simulink model "gm_mandelbrot_fpga"  (R2019b)
settings: Solver=FixedStepDiscrete  StartTime=0.0  StopTime=33.5e-3  FixedStep=0.5*Ts  RelTol=1e-3  EnableMultiTasking=on
undefined symbols (not defined in the file or in its folder): BUTTON_CLOCK_DIV, BUTTON_DEBOUNCE, BUTTON_POLLING, LUT_BLUE, LUT_GREEN, LUT_RED, MAX_ITERATIONS, PIXEL_TIME, TRASLATION_FACTOR, Ts, VGA_HORIZONTAL_BACK_PORCH, VGA_HORIZONTAL_FRONT_PORCH, VGA_HORIZONTAL_RESOLUTION, VGA_HORIZONTAL_SYNC, VGA_VERTICAL_BACK_PORCH, VGA_VERTICAL_FRONT_PORCH, VGA_VERTICAL_RESOLUTION, VGA_VERTICAL_SYNC, ZOOM_FACTOR
libraries: simulink x132, hdlsllib x20, visionsinks x1
(part 1 of 9)
settings Model: Creator=sasselll  LastModifiedBy=lucas
settings SolverCC: ZeroCrossControl=DisableAll  PositivePriorityOrder=on  MinimalZcImpactIntegration=on
settings DataIOCC: SaveOutput=off  SignalLogging=off  DSMLogging=off
settings OptimizationCC: BlockReduction=off  ConditionallyExecuteInputs=off  DefaultParameterBehavior=Inlined  EnhancedBackFolding=on  PassReuseOutputArgsAs=Individual arguments  MaxStackSize=64  OptimizeBlockOrder=speed  DifferentSizesBufferReuse=on  UseRowMajorAlgorithm=on  OptimizationCustomize=off  EfficientTunableParamExpr=on
settings DebuggingCC: ReadBeforeWriteMsg=DisableAll  WriteAfterWriteMsg=DisableAll  WriteAfterReadMsg=DisableAll  AlgebraicLoopMsg=error  InheritedTsInSrcMsg=none  MultiTaskDSMMsg=none  ParameterTunabilityLossMsg=error
settings HardwareCC: ProdBitPerPointer=32  ProdBitPerSizeT=32  ProdBitPerPtrDiffT=32  ProdLargestAtomicFloat=None  ProdIntDivRoundTo=Undefined  ProdEndianess=Unspecified  ProdWordSize=32  ProdHWDeviceType=ASIC/FPGA->ASIC/FPGA  TargetBitPerPointer=64  TargetBitPerSizeT=64  TargetBitPerPtrDiffT=64  TargetLongLongMode=on  TargetIntDivRoundTo=Zero  TargetEndianess=LittleEndian  TargetWordSize=64  TargetHWDeviceType=Custom Processor->MATLAB Host Computer  ProdEqTarget=off  HardwareBoardFeatureSet=SoCBlockset
settings ModelReferenceCC: UpdateModelReferenceTargets=IfOutOfDate
settings SFSimCC: SFSimEcho=off  MATLABDynamicMemAlloc=off  CustomCodeUndefinedFunction=UseInterfaceOnly
settings RTWCC: SystemTargetFile=ert.tlc  TemplateMakefile=ert_default_tmf  GenerateReport=on  IncludeHyperlinkInReport=on  LaunchReport=on  GenerateTraceInfo=on  GenerateTraceReport=on  GenerateTraceReportSl=on  GenerateTraceReportSf=on  GenerateTraceReportEml=on
settings CodeAppCC: ForceParamTrailComments=on  IgnoreCustomStorageClasses=off  OperatorAnnotations=on  SimulinkDataObjDesc=on  SFDataObjDesc=on  InsertBlockDesc=on
settings ERTTargetCC: InlinedParameterPlacement=NonHierarchical  ERTCustomFileTemplate=example_file_process.tlc

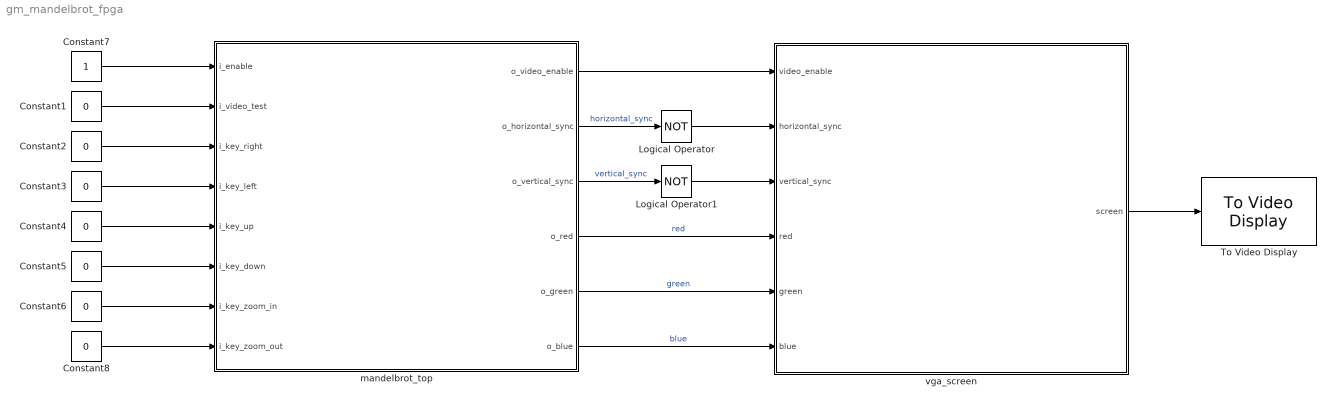
== system gm_mandelbrot_fpga ==
  Constant{1..6,8} (7 alike) : Constant  Value=0  OutDataTypeStr=boolean  SampleTime=Ts
  Constant7 : Constant  OutDataTypeStr=boolean  SampleTime=Ts
  Logical Operator : Logic  Operator=NOT  IconShape=distinctive  AllPortsSameDT=off  OutDataTypeStr=boolean
  Logical Operator1 : Logic  Operator=NOT  IconShape=distinctive  AllPortsSameDT=off  OutDataTypeStr=boolean
  To Video Display : visionsinks/To Video Display  windowSizeMode=Normal  openAtMdlStart=on  fullScreen=off  videoWindowX=810  videoWindowY=390  saveWindowSize=off  videoWindowWidth=787  videoWindowHeight=554  inputColorFormat=RGB  inputType=Obsolete  imagePorts=One multidimensional signal  OutputDevice=On-screen video monitor  dataOrg=Column-major  isWindowOpen=off
      settings: SourceProductName=Computer Vision Toolbox
  mandelbrot_top : Subsystem
  vga_screen : Subsystem
  wires:
  Constant8/1 -> mandelbrot_top/8(i_key_zoom_out)
  Constant6/1 -> mandelbrot_top/7(i_key_zoom_in)
  Constant5/1 -> mandelbrot_top/6(i_key_down)
  Constant4/1 -> mandelbrot_top/5(i_key_up)
  Constant3/1 -> mandelbrot_top/4(i_key_left)
  Constant2/1 -> mandelbrot_top/3(i_key_right)
  Logical Operator1/1 -> vga_screen/3("vertical_sync ")
  mandelbrot_top/3(o_vertical_sync) -> Logical Operator1/1  "vertical_sync"
  Logical Operator/1 -> vga_screen/2("horizontal_sync ")
  mandelbrot_top/2("o_horizontal_sync ") -> Logical Operator/1  "horizontal_sync"
  Constant1/1 -> mandelbrot_top/2(i_video_test)
  mandelbrot_top/1(o_video_enable) -> vga_screen/1("video_enable ")
  vga_screen/1(screen) -> To Video Display/1
  mandelbrot_top/6(o_blue) -> vga_screen/6(blue)  "blue"
  mandelbrot_top/5(o_green) -> vga_screen/5(green)  "green"
  mandelbrot_top/4(o_red) -> vga_screen/4(red)  "red"
  Constant7/1 -> mandelbrot_top/1(i_enable)

== system gm_mandelbrot_fpga/mandelbrot_top ==
  i_enable : Inport  OutDataTypeStr=boolean  PortDimensions=1  SampleTime=1.35e-08
  i_video_test : Inport  Port=2  OutDataTypeStr=boolean  PortDimensions=1  SampleTime=1.35e-08
  i_key_right : Inport  Port=3  OutDataTypeStr=boolean  PortDimensions=1  SampleTime=1.35e-08
  i_key_left : Inport  Port=4  OutDataTypeStr=boolean  PortDimensions=1  SampleTime=1.35e-08
  i_key_up : Inport  Port=5  OutDataTypeStr=boolean  PortDimensions=1  SampleTime=1.35e-08
  i_key_down : Inport  Port=6  OutDataTypeStr=boolean  PortDimensions=1  SampleTime=1.35e-08
  i_key_zoom_in : Inport  Port=7  OutDataTypeStr=boolean  PortDimensions=1  SampleTime=1.35e-08
  i_key_zoom_out : Inport  Port=8  OutDataTypeStr=boolean  PortDimensions=1  SampleTime=1.35e-08
  Compare To Constant : simulink/Logic and Bit Operations/Compare To Constant  relop===  const=BUTTON_CLOCK_DIV  OutDataTypeStr=boolean
  Constant : Constant  Value=BUTTON_DEBOUNCE  OutDataTypeStr=uint8  SampleTime=-1
  HDL Counter : hdlsllib/Sources/HDL Counter  CountType=Count limited  CountInit=0  CountStep=1  CountMax=BUTTON_CLOCK_DIV  CountFromType=Initial value  CountFrom=0  CountResetPort=off  CountLoadPort=off  CountEnbPort=off  CountDirPort=off  CountDataType=Unsigned  CountWordLen=17  CountFracLen=0  CountSampTime=Ts
      settings: SourceProductName=Simulink
  enable_deglitch : Subsystem
  "keyboard_handler " : Subsystem
  mandelbrot_core : Subsystem
  video_test_deglitch : Subsystem
  o_video_enable : Outport  VectorParamsAs1DForOutWhenUnconnected=off
  "o_horizontal_sync " : Outport  Port=2  VectorParamsAs1DForOutWhenUnconnected=off
  o_vertical_sync : Outport  Port=3  VectorParamsAs1DForOutWhenUnconnected=off
  o_red : Outport  Port=4  VectorParamsAs1DForOutWhenUnconnected=off
  o_green : Outport  Port=5  VectorParamsAs1DForOutWhenUnconnected=off
  o_blue : Outport  Port=6  VectorParamsAs1DForOutWhenUnconnected=off
  wires:
  i_enable/1 -> enable_deglitch/1(in)
  i_video_test/1 -> video_test_deglitch/1(in)
  i_key_right/1 -> "keyboard_handler "/1(right)
  i_key_left/1 -> "keyboard_handler "/2(left)
  i_key_up/1 -> "keyboard_handler "/3(up)
  i_key_down/1 -> "keyboard_handler "/4(down)
  i_key_zoom_in/1 -> "keyboard_handler "/5(zoom_in)
  i_key_zoom_out/1 -> "keyboard_handler "/6(zoom_out)
  Compare To Constant/1 -> video_test_deglitch/3("enable "), enable_deglitch/3("enable "), "keyboard_handler "/8(deglitch_enable)
  Constant/1 -> video_test_deglitch/2(threshold), enable_deglitch/2(threshold), "keyboard_handler "/7("deglitch_threshold ")
  HDL Counter/1 -> Compare To Constant/1
  enable_deglitch/1(out) -> mandelbrot_core/4(enable)
  "keyboard_handler "/1(zoom) -> mandelbrot_core/1(zoom)
  "keyboard_handler "/2(horizontal_offset) -> mandelbrot_core/2("horizontal_offset ")
  "keyboard_handler "/3(vertical_offset) -> mandelbrot_core/3("vertical_offset ")
  mandelbrot_core/1(video_enable) -> o_video_enable/1
  mandelbrot_core/2(horizontal_sync) -> "o_horizontal_sync "/1
  mandelbrot_core/3(vertical_sync) -> o_vertical_sync/1
  mandelbrot_core/4(red) -> o_red/1
  mandelbrot_core/5(green) -> o_green/1
  mandelbrot_core/6(blue) -> o_blue/1
  video_test_deglitch/1(out) -> mandelbrot_core/5(video_test)

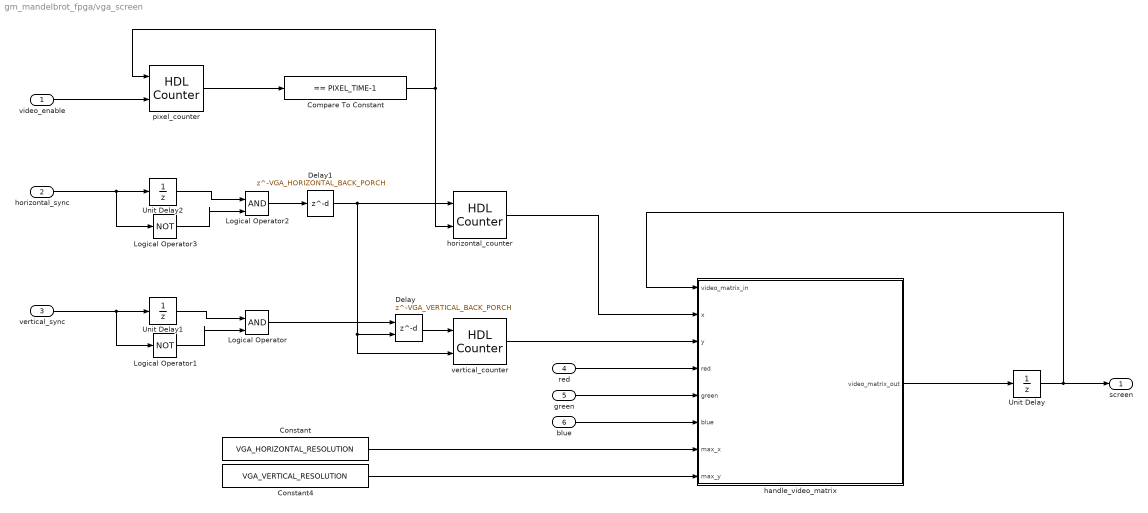
== system gm_mandelbrot_fpga/vga_screen ==
  "video_enable " : Inport
  "horizontal_sync " : Inport  Port=2
  "vertical_sync " : Inport  Port=3
  red : Inport  Port=4
  green : Inport  Port=5
  blue : Inport  Port=6
  Compare To Constant : simulink/Logic and Bit Operations/Compare To Constant  relop===  const=PIXEL_TIME-1  OutDataTypeStr=boolean
  Constant : Constant  Value=VGA_HORIZONTAL_RESOLUTION  SampleTime=-1
  Constant4 : Constant  Value=VGA_VERTICAL_RESOLUTION  SampleTime=-1
  Delay : Delay  DelayLength=VGA_VERTICAL_BACK_PORCH  InitialCondition=0  ShowEnablePort=on
      settings: InputPortMap=u0,e6
  Delay1 : Delay  DelayLength=VGA_HORIZONTAL_BACK_PORCH  InitialCondition=0
  Logical Operator : Logic  IconShape=distinctive  AllPortsSameDT=off  OutDataTypeStr=boolean
  Logical Operator1 : Logic  Operator=NOT  IconShape=distinctive  AllPortsSameDT=off  OutDataTypeStr=boolean
  Logical Operator2 : Logic  IconShape=distinctive  AllPortsSameDT=off  OutDataTypeStr=boolean
  Logical Operator3 : Logic  Operator=NOT  IconShape=distinctive  AllPortsSameDT=off  OutDataTypeStr=boolean
  Unit Delay : UnitDelay  SampleTime=-1  HasFrameUpgradeWarning=on
  Unit Delay1 : UnitDelay  SampleTime=-1  HasFrameUpgradeWarning=on
  Unit Delay2 : UnitDelay  SampleTime=-1  HasFrameUpgradeWarning=on
  handle_video_matrix : MATLAB Function  TreatAsAtomicUnit=on
  horizontal_counter : hdlsllib/Sources/HDL Counter  CountType=Free running  CountInit=1  CountStep=1  CountMax=25  CountFromType=Initial value  CountFrom=1  CountResetPort=on  CountLoadPort=off  CountEnbPort=on  CountDirPort=off  CountDataType=Unsigned  CountWordLen=16  CountFracLen=0  CountSampTime=1
      settings: SourceProductName=Simulink
  "pixel_counter " : hdlsllib/Sources/HDL Counter  CountType=Free running  CountInit=0  CountStep=1  CountMax=PIXEL_TIME  CountFromType=Initial value  CountFrom=0  CountResetPort=on  CountLoadPort=off  CountEnbPort=on  CountDirPort=off  CountDataType=Unsigned  CountWordLen=8  CountFracLen=0  CountSampTime=Ts
      settings: SourceProductName=Simulink
  vertical_counter : hdlsllib/Sources/HDL Counter  CountType=Free running  CountInit=1  CountStep=1  CountMax=25  CountFromType=Initial value  CountFrom=1  CountResetPort=on  CountLoadPort=off  CountEnbPort=on  CountDirPort=off  CountDataType=Unsigned  CountWordLen=16  CountFracLen=0  CountSampTime=1
      settings: SourceProductName=Simulink
  screen : Outport  PortDimensions=[VGA_VERTICAL_RESOLUTION VGA_HORIZONTAL_RESOLUTION 3]  VectorParamsAs1DForOutWhenUnconnected=off
  wires:
  "video_enable "/1 -> "pixel_counter "/2
  Delay1/1 -> vertical_counter/2, Delay/2, horizontal_counter/1
  Logical Operator2/1 -> Delay1/1
  Delay/1 -> vertical_counter/1
  Logical Operator/1 -> Delay/1
  Unit Delay1/1 -> Logical Operator/1
  Logical Operator1/1 -> Logical Operator/2
  Logical Operator3/1 -> Logical Operator2/2
  Unit Delay2/1 -> Logical Operator2/1
  Constant4/1 -> handle_video_matrix/8(max_y)
  Constant/1 -> handle_video_matrix/7(max_x)
  horizontal_counter/1 -> handle_video_matrix/2(x)
  blue/1 -> handle_video_matrix/6(blue)
  "vertical_sync "/1 -> Unit Delay1/1, Logical Operator1/1
  handle_video_matrix/1(video_matrix_out) -> Unit Delay/1
  vertical_counter/1 -> handle_video_matrix/3(y)
  green/1 -> handle_video_matrix/5(green)
  red/1 -> handle_video_matrix/4(red)
  Unit Delay/1 -> handle_video_matrix/1(video_matrix_in), screen/1
  Compare To Constant/1 -> horizontal_counter/2, "pixel_counter "/1
  "horizontal_sync "/1 -> Unit Delay2/1, Logical Operator3/1
  "pixel_counter "/1 -> Compare To Constant/1

== system gm_mandelbrot_fpga/mandelbrot_top/enable_deglitch ==
  in : Inport  OutDataTypeStr=boolean  SampleTime=1.35e-08
  threshold : Inport  Port=2  OutDataTypeStr=uint8  SampleTime=1.35e-08
  "enable " : Inport  Port=3  OutDataTypeStr=boolean  SampleTime=1.35e-08
  HDL Counter : hdlsllib/Sources/HDL Counter  CountType=Free running  CountInit=0  CountStep=1  CountMax=25  CountFromType=Initial value  CountFrom=0  CountResetPort=on  CountLoadPort=off  CountEnbPort=on  CountDirPort=off  CountDataType=Unsigned  CountWordLen=8  CountFracLen=0  CountSampTime=1
      settings: SourceProductName=Simulink
  Logical Operator : Logic  Operator=NOT  IconShape=distinctive  AllPortsSameDT=off  OutDataTypeStr=boolean
  Logical Operator1 : Logic  Inputs=3  IconShape=distinctive  AllPortsSameDT=off  OutDataTypeStr=boolean
  Logical Operator2 : Logic  Operator=NOT  IconShape=distinctive  AllPortsSameDT=off  OutDataTypeStr=boolean
  Relational Operator : RelationalOperator  Operator=<  OutDataTypeStr=boolean  RndMeth=Nearest
  out : Outport
  wires:
  in/1 -> Logical Operator1/1, Logical Operator/1
  threshold/1 -> Relational Operator/2
  "enable "/1 -> Logical Operator1/3
  HDL Counter/1 -> Relational Operator/1
  Logical Operator/1 -> HDL Counter/1
  Logical Operator1/1 -> HDL Counter/2
  Logical Operator2/1 -> out/1
  Relational Operator/1 -> Logical Operator2/1, Logical Operator1/2

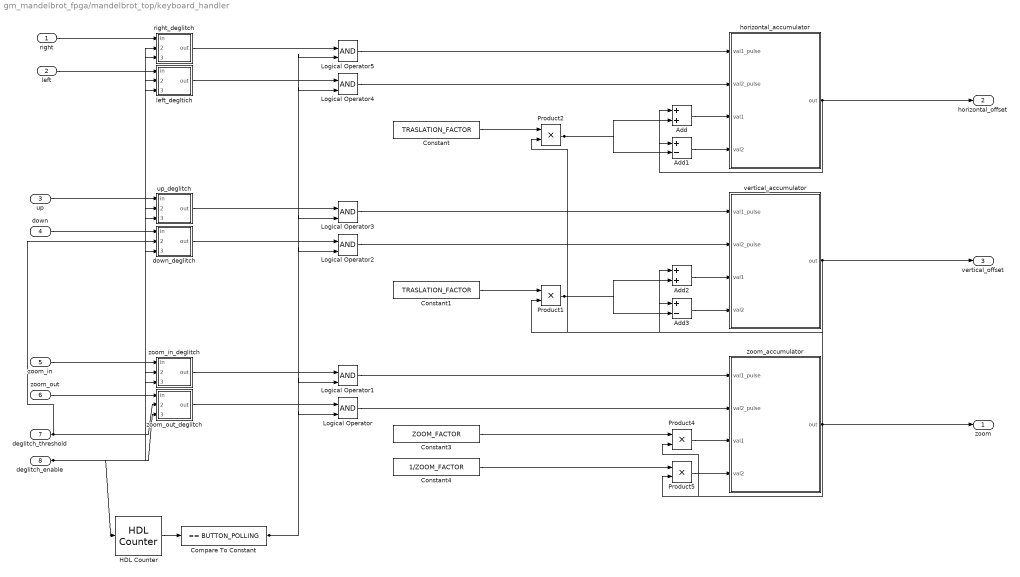
== system gm_mandelbrot_fpga/mandelbrot_top/keyboard_handler  ==
  right : Inport  OutDataTypeStr=boolean  PortDimensions=1  SampleTime=1.35e-08
  left : Inport  Port=2  OutDataTypeStr=boolean  PortDimensions=1  SampleTime=1.35e-08
  up : Inport  Port=3  OutDataTypeStr=boolean  PortDimensions=1  SampleTime=1.35e-08
  down : Inport  Port=4  OutDataTypeStr=boolean  PortDimensions=1  SampleTime=1.35e-08
  zoom_in : Inport  Port=5  OutDataTypeStr=boolean  PortDimensions=1  SampleTime=1.35e-08
  zoom_out : Inport  Port=6  OutDataTypeStr=boolean  PortDimensions=1  SampleTime=1.35e-08
  "deglitch_threshold " : Inport  Port=7  OutDataTypeStr=uint8  PortDimensions=1  SampleTime=1.35e-08
  deglitch_enable : Inport  Port=8  OutDataTypeStr=boolean  PortDimensions=1  SampleTime=1.35e-08
  Add : Sum
  Add1 : Sum  Inputs=+-
  Add2 : Sum
  Add3 : Sum  Inputs=+-  OutDataTypeStr=Inherit: Same as first input
  Compare To Constant : simulink/Logic and Bit Operations/Compare To Constant  relop===  const=BUTTON_POLLING  OutDataTypeStr=boolean
  Constant : Constant  Value=TRASLATION_FACTOR  OutDataTypeStr=Inherit: Inherit via back propagation  SampleTime=-1
  Constant1 : Constant  Value=TRASLATION_FACTOR  OutDataTypeStr=Z_BUS_TYPE  SampleTime=-1
  Constant3 : Constant  Value=ZOOM_FACTOR  OutDataTypeStr=Z_BUS_TYPE  SampleTime=-1
  Constant4 : Constant  Value=1/ZOOM_FACTOR  OutDataTypeStr=Z_BUS_TYPE  SampleTime=-1
  HDL Counter : hdlsllib/Sources/HDL Counter  CountType=Count limited  CountInit=0  CountStep=1  CountMax=BUTTON_POLLING  CountFromType=Initial value  CountFrom=0  CountResetPort=off  CountLoadPort=off  CountEnbPort=on  CountDirPort=off  CountDataType=Unsigned  CountWordLen=8  CountFracLen=0  CountSampTime=1
      settings: SourceProductName=Simulink
  Logical Operator{,1..5} (6 alike) : Logic  IconShape=distinctive  AllPortsSameDT=off  OutDataTypeStr=boolean
  Product{1..2,4..5} (4 alike) : Product  OutDataTypeStr=Inherit: Same as first input
  "down_deglitch " : Subsystem
  horizontal_accumulator : Subsystem
  left_degltich : Subsystem
  right_deglitch : Subsystem
  up_deglitch : Subsystem
  vertical_accumulator : Subsystem
  zoom_accumulator : Subsystem
  zoom_in_deglitch : Subsystem
  zoom_out_deglitch : Subsystem
  zoom : Outport  OutDataTypeStr=Z_BUS_TYPE
  horizontal_offset : Outport  Port=2  OutDataTypeStr=Z_BUS_TYPE
  vertical_offset : Outport  Port=3  OutDataTypeStr=Z_BUS_TYPE
  wires:
  right/1 -> right_deglitch/1(in)
  left/1 -> left_degltich/1(in)
  up/1 -> up_deglitch/1(in)
  down/1 -> "down_deglitch "/1(in)
  zoom_in/1 -> zoom_in_deglitch/1(in)
  zoom_out/1 -> zoom_out_deglitch/1(in)
  "deglitch_threshold "/1 -> "down_deglitch "/2(threshold), right_deglitch/2(threshold), left_degltich/2(threshold), up_deglitch/2(threshold), zoom_in_deglitch/2(threshold), zoom_out_deglitch/2(threshold)
  deglitch_enable/1 -> HDL Counter/1, zoom_out_deglitch/3("enable "), up_deglitch/3("enable "), right_deglitch/3("enable "), left_degltich/3("enable "), "down_deglitch "/3("enable "), zoom_in_deglitch/3("enable ")
  Add/1 -> horizontal_accumulator/3(val1)
  Add1/1 -> horizontal_accumulator/4(val2)
  Add2/1 -> vertical_accumulator/3(val1)
  Add3/1 -> vertical_accumulator/4(val2)
  Compare To Constant/1 -> Logical Operator5/2, Logical Operator4/2, Logical Operator3/2, Logical Operator2/2, Logical Operator1/2, Logical Operator/2
  Constant/1 -> Product2/1
  Constant1/1 -> Product1/1
  Constant3/1 -> Product4/1
  Constant4/1 -> Product5/1
  HDL Counter/1 -> Compare To Constant/1
  Logical Operator/1 -> zoom_accumulator/2(val2_pulse)
  Logical Operator1/1 -> zoom_accumulator/1(val1_pulse)
  Logical Operator2/1 -> vertical_accumulator/2(val2_pulse)
  Logical Operator3/1 -> vertical_accumulator/1(val1_pulse)
  Logical Operator4/1 -> horizontal_accumulator/2(val2_pulse)
  Logical Operator5/1 -> horizontal_accumulator/1(val1_pulse)
  Product1/1 -> Add3/2, Add2/2
  Product2/1 -> Add1/2, Add/2
  Product4/1 -> zoom_accumulator/3(val1)
  Product5/1 -> zoom_accumulator/4(val2)
  "down_deglitch "/1(out) -> Logical Operator2/1
  horizontal_accumulator/1(out) -> Add1/1, Add/1, horizontal_offset/1
  left_degltich/1(out) -> Logical Operator4/1
  right_deglitch/1(out) -> Logical Operator5/1
  up_deglitch/1(out) -> Logical Operator3/1
  vertical_accumulator/1(out) -> Add3/1, Add2/1, vertical_offset/1
  zoom_accumulator/1(out) -> Product5/2, Product4/2, Product2/2, Product1/2, zoom/1
  zoom_in_deglitch/1(out) -> Logical Operator1/1
  zoom_out_deglitch/1(out) -> Logical Operator/1

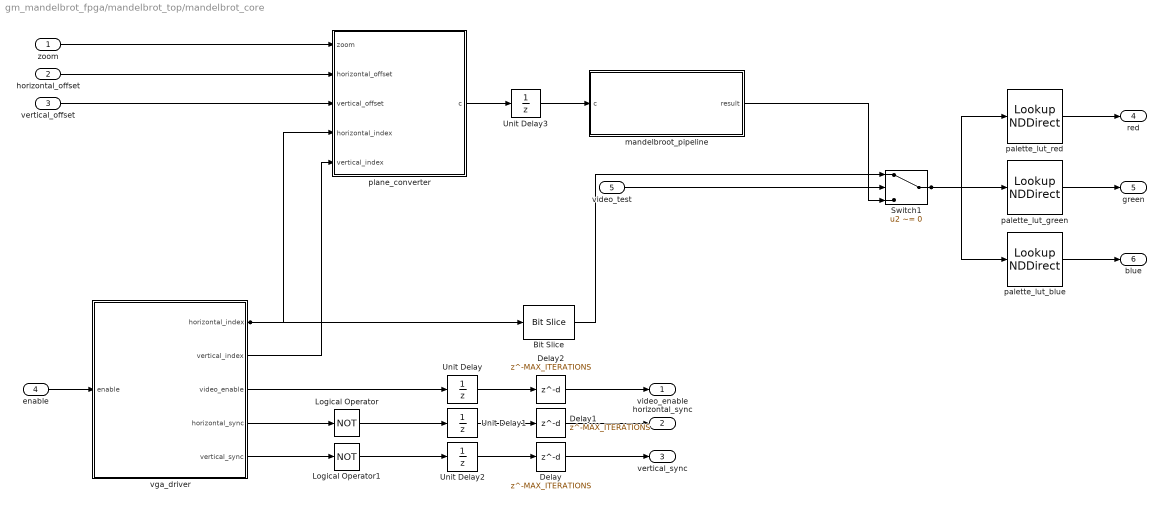
== system gm_mandelbrot_fpga/mandelbrot_top/mandelbrot_core ==
  zoom : Inport  OutDataTypeStr=fixdt(1, 18, 15)  PortDimensions=1  SampleTime=1.35e-08
  "horizontal_offset " : Inport  Port=2  OutDataTypeStr=fixdt(1, 18, 15)  PortDimensions=1  SampleTime=1.35e-08
  "vertical_offset " : Inport  Port=3  OutDataTypeStr=fixdt(1, 18, 15)  PortDimensions=1  SampleTime=1.35e-08
  enable : Inport  Port=4  OutDataTypeStr=boolean  PortDimensions=1  SampleTime=1.35e-08
  video_test : Inport  Port=5  OutDataTypeStr=boolean  PortDimensions=1  SampleTime=1.35e-08
  Bit Slice : hdlsllib/Logic and Bit Operations/Bit Slice  lidx=6  ridx=0
      settings: SourceProductName=Simulink  SourceProductBaseCode=SL
  Delay : Delay  DelayLength=MAX_ITERATIONS
  Delay1 : Delay  DelayLength=MAX_ITERATIONS
  Delay2 : Delay  DelayLength=MAX_ITERATIONS
  Logical Operator : Logic  Operator=NOT  IconShape=distinctive  AllPortsSameDT=off  OutDataTypeStr=boolean
  Logical Operator1 : Logic  Operator=NOT  IconShape=distinctive  AllPortsSameDT=off  OutDataTypeStr=boolean
  Switch1 : Switch  Criteria=u2 ~= 0
  Unit Delay{,1..3} (4 alike) : UnitDelay  SampleTime=-1  HasFrameUpgradeWarning=on
  mandelbroot_pipeline : Subsystem
  "palette_lut_blue  " : LookupNDDirect  NumberOfTableDimensions=1  Table=LUT_BLUE  DiagnosticForOutOfRangeInput=Error
  "palette_lut_green " : LookupNDDirect  NumberOfTableDimensions=1  Table=LUT_GREEN  DiagnosticForOutOfRangeInput=Error
  "palette_lut_red " : LookupNDDirect  NumberOfTableDimensions=1  Table=LUT_RED  DiagnosticForOutOfRangeInput=Error
  "plane_converter " : Subsystem
  vga_driver : Subsystem
  video_enable : Outport  VectorParamsAs1DForOutWhenUnconnected=off
  horizontal_sync : Outport  Port=2  VectorParamsAs1DForOutWhenUnconnected=off
  vertical_sync : Outport  Port=3  VectorParamsAs1DForOutWhenUnconnected=off
  red : Outport  Port=4  VectorParamsAs1DForOutWhenUnconnected=off
  green : Outport  Port=5  VectorParamsAs1DForOutWhenUnconnected=off
  blue : Outport  Port=6  VectorParamsAs1DForOutWhenUnconnected=off
  wires:
  zoom/1 -> "plane_converter "/1(zoom)
  "horizontal_offset "/1 -> "plane_converter "/2("horizontal_offset ")
  "vertical_offset "/1 -> "plane_converter "/3("vertical_offset ")
  enable/1 -> vga_driver/1("enable ")
  video_test/1 -> Switch1/2
  Bit Slice/1 -> Switch1/1
  Delay/1 -> vertical_sync/1
  Delay1/1 -> horizontal_sync/1
  Delay2/1 -> video_enable/1
  Logical Operator/1 -> Unit Delay1/1
  Logical Operator1/1 -> Unit Delay2/1
  Switch1/1 -> "palette_lut_red "/1, "palette_lut_green "/1, "palette_lut_blue  "/1
  Unit Delay/1 -> Delay2/1
  Unit Delay1/1 -> Delay1/1
  Unit Delay2/1 -> Delay/1
  Unit Delay3/1 -> mandelbroot_pipeline/1(c)
  mandelbroot_pipeline/1(result) -> Switch1/3
  "palette_lut_blue  "/1 -> blue/1
  "palette_lut_green "/1 -> green/1
  "palette_lut_red "/1 -> red/1
  "plane_converter "/1(c) -> Unit Delay3/1
  vga_driver/1(horizontal_index) -> Bit Slice/1, "plane_converter "/4("horizontal_index ")
  vga_driver/2(vertical_index) -> "plane_converter "/5("vertical_index ")
  vga_driver/3("video_enable ") -> Unit Delay/1
  vga_driver/4(horizontal_sync) -> Logical Operator/1
  vga_driver/5("vertical_sync ") -> Logical Operator1/1

== system gm_mandelbrot_fpga/mandelbrot_top/video_test_deglitch ==
  in : Inport  OutDataTypeStr=boolean  SampleTime=1.35e-08
  threshold : Inport  Port=2  OutDataTypeStr=uint8  SampleTime=1.35e-08
  "enable " : Inport  Port=3  OutDataTypeStr=boolean  SampleTime=1.35e-08
  HDL Counter : hdlsllib/Sources/HDL Counter  CountType=Free running  CountInit=0  CountStep=1  CountMax=25  CountFromType=Initial value  CountFrom=0  CountResetPort=on  CountLoadPort=off  CountEnbPort=on  CountDirPort=off  CountDataType=Unsigned  CountWordLen=8  CountFracLen=0  CountSampTime=1
      settings: SourceProductName=Simulink
  Logical Operator : Logic  Operator=NOT  IconShape=distinctive  AllPortsSameDT=off  OutDataTypeStr=boolean
  Logical Operator1 : Logic  Inputs=3  IconShape=distinctive  AllPortsSameDT=off  OutDataTypeStr=boolean
  Logical Operator2 : Logic  Operator=NOT  IconShape=distinctive  AllPortsSameDT=off  OutDataTypeStr=boolean
  Relational Operator : RelationalOperator  Operator=<  OutDataTypeStr=boolean  RndMeth=Nearest
  out : Outport
  wires:
  in/1 -> Logical Operator1/1, Logical Operator/1
  threshold/1 -> Relational Operator/2
  "enable "/1 -> Logical Operator1/3
  HDL Counter/1 -> Relational Operator/1
  Logical Operator/1 -> HDL Counter/1
  Logical Operator1/1 -> HDL Counter/2
  Logical Operator2/1 -> out/1
  Relational Operator/1 -> Logical Operator2/1, Logical Operator1/2

== system gm_mandelbrot_fpga/mandelbrot_top/keyboard_handler /down_deglitch  ==
  in : Inport  OutDataTypeStr=boolean  SampleTime=1.35e-08
  threshold : Inport  Port=2  OutDataTypeStr=uint8  SampleTime=1.35e-08
  "enable " : Inport  Port=3  OutDataTypeStr=boolean  SampleTime=1.35e-08
  HDL Counter : hdlsllib/Sources/HDL Counter  CountType=Free running  CountInit=0  CountStep=1  CountMax=25  CountFromType=Initial value  CountFrom=0  CountResetPort=on  CountLoadPort=off  CountEnbPort=on  CountDirPort=off  CountDataType=Unsigned  CountWordLen=8  CountFracLen=0  CountSampTime=1
      settings: SourceProductName=Simulink
  Logical Operator : Logic  Operator=NOT  IconShape=distinctive  AllPortsSameDT=off  OutDataTypeStr=boolean
  Logical Operator1 : Logic  Inputs=3  IconShape=distinctive  AllPortsSameDT=off  OutDataTypeStr=boolean
  Logical Operator2 : Logic  Operator=NOT  IconShape=distinctive  AllPortsSameDT=off  OutDataTypeStr=boolean
  Relational Operator : RelationalOperator  Operator=<  OutDataTypeStr=boolean  RndMeth=Nearest
  out : Outport
  wires:
  in/1 -> Logical Operator1/1, Logical Operator/1
  threshold/1 -> Relational Operator/2
  "enable "/1 -> Logical Operator1/3
  HDL Counter/1 -> Relational Operator/1
  Logical Operator/1 -> HDL Counter/1
  Logical Operator1/1 -> HDL Counter/2
  Logical Operator2/1 -> out/1
  Relational Operator/1 -> Logical Operator2/1, Logical Operator1/2

== system gm_mandelbrot_fpga/mandelbrot_top/keyboard_handler /horizontal_accumulator ==
  val1_pulse : Inport  OutDataTypeStr=boolean  SampleTime=1.35e-08
  val2_pulse : Inport  Port=2  OutDataTypeStr=boolean  SampleTime=1.35e-08
  val1 : Inport  Port=3  OutDataTypeStr=fixdt(1, 18, 15)  SampleTime=1.35e-08
  val2 : Inport  Port=4  OutDataTypeStr=fixdt(1, 18, 15)  SampleTime=1.35e-08
  Delay1 : Delay  DelayLength=1
  Delay2 : Delay  DelayLength=1
  Logical Operator : Logic  IconShape=distinctive  AllPortsSameDT=off  OutDataTypeStr=boolean
  Logical Operator1 : Logic  Operator=NOT  IconShape=distinctive  AllPortsSameDT=off  OutDataTypeStr=boolean
  Logical Operator2 : Logic  IconShape=distinctive  AllPortsSameDT=off  OutDataTypeStr=boolean
  Logical Operator3 : Logic  Operator=NOT  IconShape=distinctive  AllPortsSameDT=off  OutDataTypeStr=boolean
  Logical Operator4 : Logic  Operator=OR  IconShape=distinctive  AllPortsSameDT=off  OutDataTypeStr=boolean
  Switch : Switch
  Unit Delay Enabled Synchronous : hdlsllib/Discrete/Unit Delay Enabled Synchronous  InitialCondition=0.0  SampleTime=-1
      settings: SourceProductName=Simulink  SourceProductBaseCode=SL
  out : Outport
  wires:
  val1_pulse/1 -> Logical Operator/2, Delay1/1
  val2_pulse/1 -> Logical Operator2/2, Delay2/1
  val1/1 -> Switch/1
  val2/1 -> Switch/3
  Delay1/1 -> Logical Operator1/1
  Delay2/1 -> Logical Operator3/1
  Logical Operator/1 -> Switch/2, Logical Operator4/1
  Logical Operator1/1 -> Logical Operator/1
  Logical Operator2/1 -> Logical Operator4/2
  Logical Operator3/1 -> Logical Operator2/1
  Logical Operator4/1 -> Unit Delay Enabled Synchronous/2
  Switch/1 -> Unit Delay Enabled Synchronous/1
  Unit Delay Enabled Synchronous/1 -> out/1

== system gm_mandelbrot_fpga/mandelbrot_top/keyboard_handler /left_degltich ==
  in : Inport  OutDataTypeStr=boolean  SampleTime=1.35e-08
  threshold : Inport  Port=2  OutDataTypeStr=uint8  SampleTime=1.35e-08
  "enable " : Inport  Port=3  OutDataTypeStr=boolean  SampleTime=1.35e-08
  HDL Counter : hdlsllib/Sources/HDL Counter  CountType=Free running  CountInit=0  CountStep=1  CountMax=25  CountFromType=Initial value  CountFrom=0  CountResetPort=on  CountLoadPort=off  CountEnbPort=on  CountDirPort=off  CountDataType=Unsigned  CountWordLen=8  CountFracLen=0  CountSampTime=1
      settings: SourceProductName=Simulink
  Logical Operator : Logic  Operator=NOT  IconShape=distinctive  AllPortsSameDT=off  OutDataTypeStr=boolean
  Logical Operator1 : Logic  Inputs=3  IconShape=distinctive  AllPortsSameDT=off  OutDataTypeStr=boolean
  Logical Operator2 : Logic  Operator=NOT  IconShape=distinctive  AllPortsSameDT=off  OutDataTypeStr=boolean
  Relational Operator : RelationalOperator  Operator=<  OutDataTypeStr=boolean  RndMeth=Nearest
  out : Outport
  wires:
  in/1 -> Logical Operator1/1, Logical Operator/1
  threshold/1 -> Relational Operator/2
  "enable "/1 -> Logical Operator1/3
  HDL Counter/1 -> Relational Operator/1
  Logical Operator/1 -> HDL Counter/1
  Logical Operator1/1 -> HDL Counter/2
  Logical Operator2/1 -> out/1
  Relational Operator/1 -> Logical Operator2/1, Logical Operator1/2

== system gm_mandelbrot_fpga/mandelbrot_top/keyboard_handler /right_deglitch ==
  in : Inport  OutDataTypeStr=boolean  SampleTime=1.35e-08
  threshold : Inport  Port=2  OutDataTypeStr=uint8  SampleTime=1.35e-08
  "enable " : Inport  Port=3  OutDataTypeStr=boolean  SampleTime=1.35e-08
  HDL Counter : hdlsllib/Sources/HDL Counter  CountType=Free running  CountInit=0  CountStep=1  CountMax=25  CountFromType=Initial value  CountFrom=0  CountResetPort=on  CountLoadPort=off  CountEnbPort=on  CountDirPort=off  CountDataType=Unsigned  CountWordLen=8  CountFracLen=0  CountSampTime=1
      settings: SourceProductName=Simulink
  Logical Operator : Logic  Operator=NOT  IconShape=distinctive  AllPortsSameDT=off  OutDataTypeStr=boolean
  Logical Operator1 : Logic  Inputs=3  IconShape=distinctive  AllPortsSameDT=off  OutDataTypeStr=boolean
  Logical Operator2 : Logic  Operator=NOT  IconShape=distinctive  AllPortsSameDT=off  OutDataTypeStr=boolean
  Relational Operator : RelationalOperator  Operator=<  OutDataTypeStr=boolean  RndMeth=Nearest
  out : Outport
  wires:
  in/1 -> Logical Operator1/1, Logical Operator/1
  threshold/1 -> Relational Operator/2
  "enable "/1 -> Logical Operator1/3
  HDL Counter/1 -> Relational Operator/1
  Logical Operator/1 -> HDL Counter/1
  Logical Operator1/1 -> HDL Counter/2
  Logical Operator2/1 -> out/1
  Relational Operator/1 -> Logical Operator2/1, Logical Operator1/2

== system gm_mandelbrot_fpga/mandelbrot_top/keyboard_handler /up_deglitch ==
  in : Inport  OutDataTypeStr=boolean  SampleTime=1.35e-08
  threshold : Inport  Port=2  OutDataTypeStr=uint8  SampleTime=1.35e-08
  "enable " : Inport  Port=3  OutDataTypeStr=boolean  SampleTime=1.35e-08
  HDL Counter : hdlsllib/Sources/HDL Counter  CountType=Free running  CountInit=0  CountStep=1  CountMax=25  CountFromType=Initial value  CountFrom=0  CountResetPort=on  CountLoadPort=off  CountEnbPort=on  CountDirPort=off  CountDataType=Unsigned  CountWordLen=8  CountFracLen=0  CountSampTime=1
      settings: SourceProductName=Simulink
  Logical Operator : Logic  Operator=NOT  IconShape=distinctive  AllPortsSameDT=off  OutDataTypeStr=boolean
  Logical Operator1 : Logic  Inputs=3  IconShape=distinctive  AllPortsSameDT=off  OutDataTypeStr=boolean
  Logical Operator2 : Logic  Operator=NOT  IconShape=distinctive  AllPortsSameDT=off  OutDataTypeStr=boolean
  Relational Operator : RelationalOperator  Operator=<  OutDataTypeStr=boolean  RndMeth=Nearest
  out : Outport
  wires:
  in/1 -> Logical Operator1/1, Logical Operator/1
  threshold/1 -> Relational Operator/2
  "enable "/1 -> Logical Operator1/3
  HDL Counter/1 -> Relational Operator/1
  Logical Operator/1 -> HDL Counter/1
  Logical Operator1/1 -> HDL Counter/2
  Logical Operator2/1 -> out/1
  Relational Operator/1 -> Logical Operator2/1, Logical Operator1/2

== system gm_mandelbrot_fpga/mandelbrot_top/keyboard_handler /vertical_accumulator ==
  val1_pulse : Inport  OutDataTypeStr=boolean  SampleTime=1.35e-08
  val2_pulse : Inport  Port=2  OutDataTypeStr=boolean  SampleTime=1.35e-08
  val1 : Inport  Port=3  OutDataTypeStr=fixdt(1, 18, 15)  SampleTime=1.35e-08
  val2 : Inport  Port=4  OutDataTypeStr=fixdt(1, 18, 15)  SampleTime=1.35e-08
  Delay1 : Delay  DelayLength=1
  Delay2 : Delay  DelayLength=1
  Logical Operator : Logic  IconShape=distinctive  AllPortsSameDT=off  OutDataTypeStr=boolean
  Logical Operator1 : Logic  Operator=NOT  IconShape=distinctive  AllPortsSameDT=off  OutDataTypeStr=boolean
  Logical Operator2 : Logic  IconShape=distinctive  AllPortsSameDT=off  OutDataTypeStr=boolean
  Logical Operator3 : Logic  Operator=NOT  IconShape=distinctive  AllPortsSameDT=off  OutDataTypeStr=boolean
  Logical Operator4 : Logic  Operator=OR  IconShape=distinctive  AllPortsSameDT=off  OutDataTypeStr=boolean
  Switch : Switch
  Unit Delay Enabled Synchronous : hdlsllib/Discrete/Unit Delay Enabled Synchronous  InitialCondition=0.0  SampleTime=-1
      settings: SourceProductName=Simulink  SourceProductBaseCode=SL
  out : Outport
  wires:
  val1_pulse/1 -> Logical Operator/2, Delay1/1
  val2_pulse/1 -> Logical Operator2/2, Delay2/1
  val1/1 -> Switch/1
  val2/1 -> Switch/3
  Delay1/1 -> Logical Operator1/1
  Delay2/1 -> Logical Operator3/1
  Logical Operator/1 -> Switch/2, Logical Operator4/1
  Logical Operator1/1 -> Logical Operator/1
  Logical Operator2/1 -> Logical Operator4/2
  Logical Operator3/1 -> Logical Operator2/1
  Logical Operator4/1 -> Unit Delay Enabled Synchronous/2
  Switch/1 -> Unit Delay Enabled Synchronous/1
  Unit Delay Enabled Synchronous/1 -> out/1

== system gm_mandelbrot_fpga/mandelbrot_top/keyboard_handler /zoom_accumulator ==
  val1_pulse : Inport  OutDataTypeStr=boolean  SampleTime=1.35e-08
  val2_pulse : Inport  Port=2  OutDataTypeStr=boolean  SampleTime=1.35e-08
  val1 : Inport  Port=3  OutDataTypeStr=fixdt(1, 18, 15)  SampleTime=1.35e-08
  val2 : Inport  Port=4  OutDataTypeStr=fixdt(1, 18, 15)  SampleTime=1.35e-08
  Delay1 : Delay  DelayLength=1
  Delay2 : Delay  DelayLength=1
  Logical Operator : Logic  IconShape=distinctive  AllPortsSameDT=off  OutDataTypeStr=boolean
  Logical Operator1 : Logic  Operator=NOT  IconShape=distinctive  AllPortsSameDT=off  OutDataTypeStr=boolean
  Logical Operator2 : Logic  IconShape=distinctive  AllPortsSameDT=off  OutDataTypeStr=boolean
  Logical Operator3 : Logic  Operator=NOT  IconShape=distinctive  AllPortsSameDT=off  OutDataTypeStr=boolean
  Logical Operator4 : Logic  Operator=OR  IconShape=distinctive  AllPortsSameDT=off  OutDataTypeStr=boolean
  Switch : Switch
  Unit Delay Enabled Synchronous : hdlsllib/Discrete/Unit Delay Enabled Synchronous  InitialCondition=1  SampleTime=-1
      settings: SourceProductName=Simulink  SourceProductBaseCode=SL
  out : Outport
  wires:
  val1_pulse/1 -> Logical Operator/2, Delay1/1
  val2_pulse/1 -> Logical Operator2/2, Delay2/1
  val1/1 -> Switch/1
  val2/1 -> Switch/3
  Delay1/1 -> Logical Operator1/1
  Delay2/1 -> Logical Operator3/1
  Logical Operator/1 -> Switch/2, Logical Operator4/1
  Logical Operator1/1 -> Logical Operator/1
  Logical Operator2/1 -> Logical Operator4/2
  Logical Operator3/1 -> Logical Operator2/1
  Logical Operator4/1 -> Unit Delay Enabled Synchronous/2
  Switch/1 -> Unit Delay Enabled Synchronous/1
  Unit Delay Enabled Synchronous/1 -> out/1

== system gm_mandelbrot_fpga/mandelbrot_top/keyboard_handler /zoom_in_deglitch ==
  in : Inport  OutDataTypeStr=boolean  SampleTime=1.35e-08
  threshold : Inport  Port=2  OutDataTypeStr=uint8  SampleTime=1.35e-08
  "enable " : Inport  Port=3  OutDataTypeStr=boolean  SampleTime=1.35e-08
  HDL Counter : hdlsllib/Sources/HDL Counter  CountType=Free running  CountInit=0  CountStep=1  CountMax=25  CountFromType=Initial value  CountFrom=0  CountResetPort=on  CountLoadPort=off  CountEnbPort=on  CountDirPort=off  CountDataType=Unsigned  CountWordLen=8  CountFracLen=0  CountSampTime=1
      settings: SourceProductName=Simulink
  Logical Operator : Logic  Operator=NOT  IconShape=distinctive  AllPortsSameDT=off  OutDataTypeStr=boolean
  Logical Operator1 : Logic  Inputs=3  IconShape=distinctive  AllPortsSameDT=off  OutDataTypeStr=boolean
  Logical Operator2 : Logic  Operator=NOT  IconShape=distinctive  AllPortsSameDT=off  OutDataTypeStr=boolean
  Relational Operator : RelationalOperator  Operator=<  OutDataTypeStr=boolean  RndMeth=Nearest
  out : Outport
  wires:
  in/1 -> Logical Operator1/1, Logical Operator/1
  threshold/1 -> Relational Operator/2
  "enable "/1 -> Logical Operator1/3
  HDL Counter/1 -> Relational Operator/1
  Logical Operator/1 -> HDL Counter/1
  Logical Operator1/1 -> HDL Counter/2
  Logical Operator2/1 -> out/1
  Relational Operator/1 -> Logical Operator2/1, Logical Operator1/2

== system gm_mandelbrot_fpga/mandelbrot_top/keyboard_handler /zoom_out_deglitch ==
  in : Inport  OutDataTypeStr=boolean  SampleTime=1.35e-08
  threshold : Inport  Port=2  OutDataTypeStr=uint8  SampleTime=1.35e-08
  "enable " : Inport  Port=3  OutDataTypeStr=boolean  SampleTime=1.35e-08
  HDL Counter : hdlsllib/Sources/HDL Counter  CountType=Free running  CountInit=0  CountStep=1  CountMax=25  CountFromType=Initial value  CountFrom=0  CountResetPort=on  CountLoadPort=off  CountEnbPort=on  CountDirPort=off  CountDataType=Unsigned  CountWordLen=8  CountFracLen=0  CountSampTime=1
      settings: SourceProductName=Simulink
  Logical Operator : Logic  Operator=NOT  IconShape=distinctive  AllPortsSameDT=off  OutDataTypeStr=boolean
  Logical Operator1 : Logic  Inputs=3  IconShape=distinctive  AllPortsSameDT=off  OutDataTypeStr=boolean
  Logical Operator2 : Logic  Operator=NOT  IconShape=distinctive  AllPortsSameDT=off  OutDataTypeStr=boolean
  Relational Operator : RelationalOperator  Operator=<  OutDataTypeStr=boolean  RndMeth=Nearest
  out : Outport
  wires:
  in/1 -> Logical Operator1/1, Logical Operator/1
  threshold/1 -> Relational Operator/2
  "enable "/1 -> Logical Operator1/3
  HDL Counter/1 -> Relational Operator/1
  Logical Operator/1 -> HDL Counter/1
  Logical Operator1/1 -> HDL Counter/2
  Logical Operator2/1 -> out/1
  Relational Operator/1 -> Logical Operator2/1, Logical Operator1/2
